simulink model "FM_recv_CIC"  (R2019a)
settings: Solver=VariableStepAuto  StartTime=0.0  StopTime=0.1  RelTol=1e-3
libraries: dspmlti4 x4, dspfdesign x2, commanapbnd3 x1
settings Model: Creator=Wunyje  LastModifiedBy=Wunyje

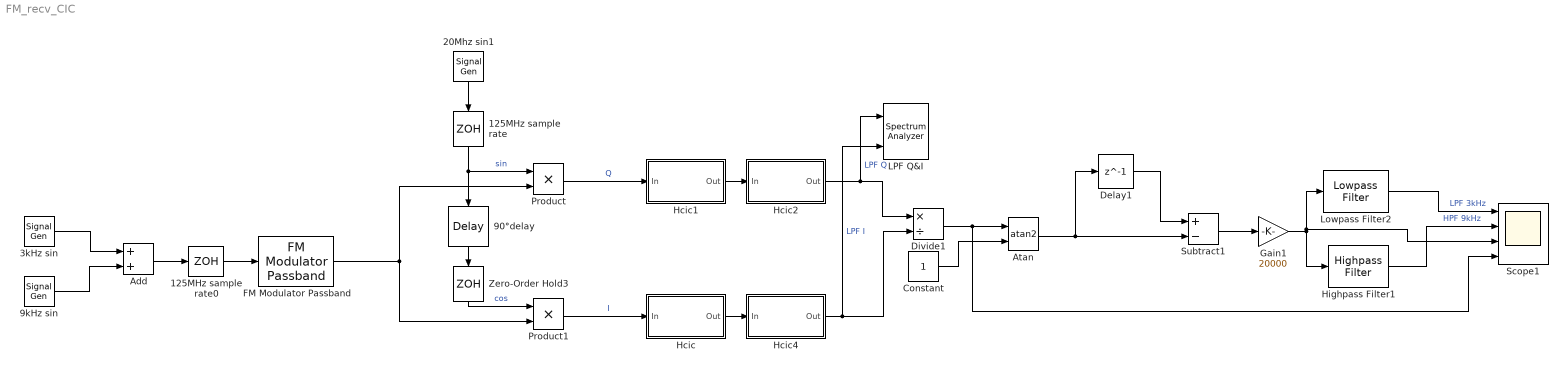
== system FM_recv_CIC ==
  125MHz sample rate : ZeroOrderHold  SampleTime=8e-9
  125MHz sample rate0 : ZeroOrderHold  SampleTime=8e-9
  20Mhz sin1 : SignalGenerator  Frequency=20e6
  3kHz sin : SignalGenerator  Frequency=3000
  90°delay : TransportDelay  DelayTime=12.5e-9
  "9kHz sin " : SignalGenerator  Frequency=9000
  Add : Sum
  Atan : Trigonometry  Operator=atan2  ApproximationMethod=CORDIC  NumberOfIterations=15
  Constant : Constant  OutDataTypeStr=fixdt(1,32,15)  SampleTime=5e-6
  Delay1 : Delay  DelayLength=1  InitialCondition=0
  Divide1 : Product  Inputs=*/  OutMin=0  OutMax=0.06  OutDataTypeStr=fixdt(1,32,15)
  FM Modulator Passband : commanapbnd3/FM Modulator Passband  Fc=20e6  Ph=0  Kc=50
      settings: SourceProductName=Communications Toolbox  SourceProductBaseCode=CM
  Gain1 : Gain  Gain=20000
  Hcic : Subsystem  Tag=BlockMethodSubSystem
  Hcic1 : Subsystem  Tag=BlockMethodSubSystem
  Hcic2 : Subsystem  Tag=BlockMethodSubSystem
  Hcic4 : Subsystem  Tag=BlockMethodSubSystem
  Highpass Filter1 : dspfdesign/Highpass Filter  FilterType=FIR  DesignForMinimumOrder=on  FilterOrder=50  StopbandFrequency=4e3  PassbandFrequency=6e3  StopbandAttenuation=80  PassbandRipple=0.1  InheritSampleRate=off  SampleRate=200e3  SimulateUsing=Interpreted execution  roundingMode=Floor  coeffsDataTypeStr=fixdt(1,16)
      settings: SourceProductName=DSP System Toolbox
  LPF Q&I : SpectrumAnalyzer  NumInputPorts=2
  Lowpass Filter2 : dspfdesign/Lowpass Filter  FilterType=FIR  DesignForMinimumOrder=on  FilterOrder=50  PassbandFrequency=5e3  StopbandFrequency=7e3  PassbandRipple=0.1  StopbandAttenuation=80  InheritSampleRate=off  SampleRate=200e3  SimulateUsing=Interpreted execution  roundingMode=Floor  coeffsDataTypeStr=fixdt(1,16)
  Product : Product
  Product1 : Product
  Scope1 : Scope  NumInputPorts=4
  Subtract1 : Sum  Inputs=+-
  Zero-Order Hold3 : ZeroOrderHold  SampleTime=8e-9
  wires:
  20Mhz sin1/1 -> 125MHz sample rate/1
  Zero-Order Hold3/1 -> Product1/1  "cos"
  90°delay/1 -> Zero-Order Hold3/1
  Product/1 -> Hcic1/1(In)  "Q"
  Product1/1 -> Hcic/1(In)  "I"
  Add/1 -> 125MHz sample rate0/1
  125MHz sample rate0/1 -> FM Modulator Passband/1
  "9kHz sin "/1 -> Add/2
  125MHz sample rate/1 -> 90°delay/1, Product/1  "sin"
  3kHz sin/1 -> Add/1
  Hcic4/1(Out) -> Divide1/2, LPF Q&I/2  "LPF I"
  Hcic2/1(Out) -> Divide1/1, LPF Q&I/1  "LPF Q"
  FM Modulator Passband/1 -> Product/2, Product1/2
  Hcic/1(Out) -> Hcic4/1(In)
  Hcic1/1(Out) -> Hcic2/1(In)
  Divide1/1 -> Atan/1, Scope1/4
  Constant/1 -> Atan/2
  Delay1/1 -> Subtract1/1
  Highpass Filter1/1 -> Scope1/2  "HPF 9kHz"
  Atan/1 -> Subtract1/2, Delay1/1
  Gain1/1 -> Lowpass Filter2/1, Scope1/3, Highpass Filter1/1
  Lowpass Filter2/1 -> Scope1/1  "LPF 3kHz"
  Subtract1/1 -> Gain1/1

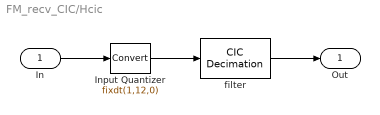
== system FM_recv_CIC/Hcic ==
  In : Inport
  Input Quantizer : DataTypeConversion  OutDataTypeStr=fixdt(1,12,0)  RndMeth=Round  SaturateOnIntegerOverflow=on
  filter : dspmlti4/CIC Decimation  filtFrom=Dialog parameters  filtobj=CICDECIM  ftype=Decimator  R=25  M=1  N=1  filterInternals=Full precision  BPS=[17 17]  FLPS=[0 0]  outputWordLength=17  outputFracLength=0  launchFVT=off  framing=Maintain input frame rate  RateOptions=Allow multirate processing
      settings: SourceProductName=DSP System Toolbox  SourceProductBaseCode=DS
  Out : Outport
  wires:
  In/1 -> Input Quantizer/1
  Input Quantizer/1 -> filter/1
  filter/1 -> Out/1

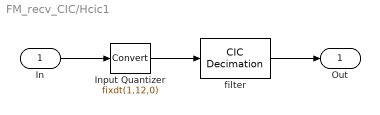
== system FM_recv_CIC/Hcic1 ==
  In : Inport
  Input Quantizer : DataTypeConversion  OutDataTypeStr=fixdt(1,12,0)  RndMeth=Round  SaturateOnIntegerOverflow=on
  filter : dspmlti4/CIC Decimation  filtFrom=Dialog parameters  filtobj=CICDECIM  ftype=Decimator  R=25  M=1  N=1  filterInternals=Full precision  BPS=[17 17]  FLPS=[0 0]  outputWordLength=17  outputFracLength=0  launchFVT=off  framing=Maintain input frame rate  RateOptions=Allow multirate processing
      settings: SourceProductName=DSP System Toolbox  SourceProductBaseCode=DS
  Out : Outport
  wires:
  In/1 -> Input Quantizer/1
  Input Quantizer/1 -> filter/1
  filter/1 -> Out/1

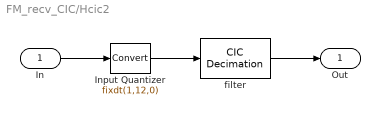
== system FM_recv_CIC/Hcic2 ==
  In : Inport
  Input Quantizer : DataTypeConversion  OutDataTypeStr=fixdt(1,12,0)  RndMeth=Round  SaturateOnIntegerOverflow=on
  filter : dspmlti4/CIC Decimation  filtFrom=Dialog parameters  filtobj=CICDECIM  ftype=Decimator  R=25  M=1  N=1  filterInternals=Full precision  BPS=[17 17]  FLPS=[0 0]  outputWordLength=17  outputFracLength=0  launchFVT=off  framing=Maintain input frame rate  RateOptions=Allow multirate processing
      settings: SourceProductName=DSP System Toolbox  SourceProductBaseCode=DS
  Out : Outport
  wires:
  In/1 -> Input Quantizer/1
  Input Quantizer/1 -> filter/1
  filter/1 -> Out/1

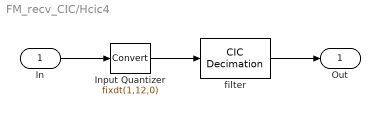
== system FM_recv_CIC/Hcic4 ==
  In : Inport
  Input Quantizer : DataTypeConversion  OutDataTypeStr=fixdt(1,12,0)  RndMeth=Round  SaturateOnIntegerOverflow=on
  filter : dspmlti4/CIC Decimation  filtFrom=Dialog parameters  filtobj=CICDECIM  ftype=Decimator  R=25  M=1  N=1  filterInternals=Full precision  BPS=[17 17]  FLPS=[0 0]  outputWordLength=17  outputFracLength=0  launchFVT=off  framing=Maintain input frame rate  RateOptions=Allow multirate processing
      settings: SourceProductName=DSP System Toolbox  SourceProductBaseCode=DS
  Out : Outport
  wires:
  In/1 -> Input Quantizer/1
  Input Quantizer/1 -> filter/1
  filter/1 -> Out/1
